simulink model "bicycle_drift_model"  (R2016a)
settings: Solver=VariableStepAuto  StartTime=0.0  StopTime=20  RelTol=1e-3
values from neighbouring files (symbols this model uses):
  a = 0.1    [setup.m]
  b = 0.155    [setup.m]
  C_alpha = 10    [setup.m]
  initial_states = [0 0 3]    [setup.m]
  Iz = 0.2    [setup.m]
  L = 0.255    [setup.m]    (also in veh_object2.m = obj_length)
  m = 5    [setup.m]
  mu = 0.2    [setup.m]
undefined symbols (not defined in the file): animation_update_interval, datetime, enable_CG_trace, enable_rearAxle_trace, plotAxisLimitMode, plotAxisLimits, save_anim_frames, vehicle_length, vehicle_width
settings Model: Creator=Cyrus  LastModifiedBy=Cyrus

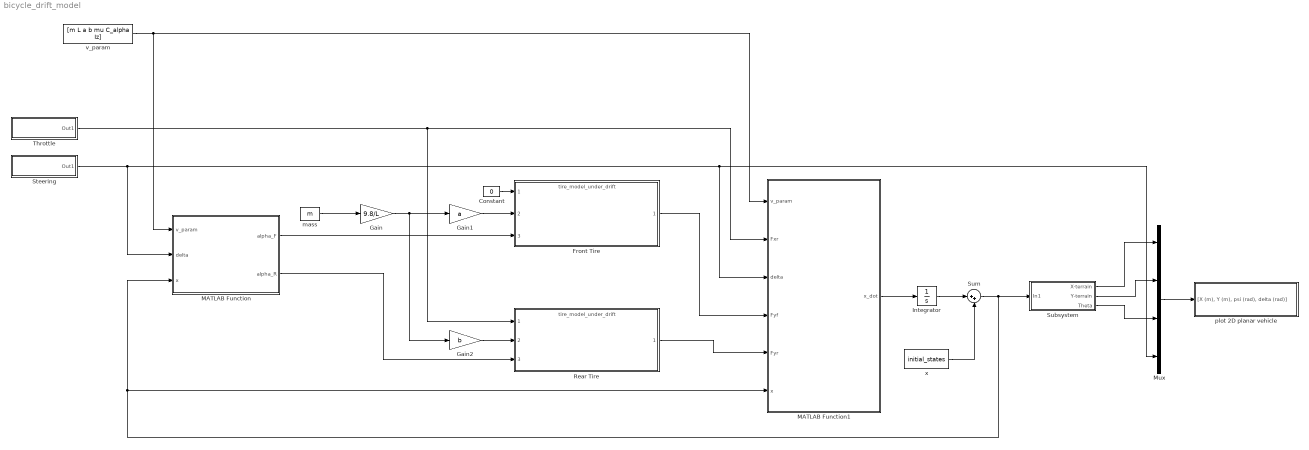
== system bicycle_drift_model ==
  Constant : Constant  Value=0
  Front Tire : ModelReference  ModelNameDialog=tire_model_under_drift.slx  SimulationMode=Normal  ModelReferenceVersion=1.21
  Gain : Gain  Gain=9.8/L
  Gain1 : Gain  Gain=a
  Gain2 : Gain  Gain=b
  Integrator : Integrator
  MATLAB Function : MATLAB Function  TreatAsAtomicUnit=on
  MATLAB Function1 : MATLAB Function  TreatAsAtomicUnit=on
  Mux : Mux
  Rear Tire : ModelReference  ModelNameDialog=tire_model_under_drift.slx  SimulationMode=Normal  ModelReferenceVersion=1.21
  Steering : Subsystem
  Subsystem : Subsystem
  Sum : Sum  Inputs=|++
  Throttle : Subsystem
  mass : Constant  Value=m
  plot 2D planar vehicle : Subsystem  mask(6DoF Animation){axisMode=plotAxisLimitMode, ax=plotAxisLimits, Ts=animation_update_interval, enable_CG_trace=enable_CG_trace, enable_rearAxle_trace=enable_rearAxle_trace, save_anim_frames=save_anim_frames, anim_frame_name_str=char(datetime('now','Format','yyyy-MM-dd_HH_mm_ss')), L=vehicle_length, W=vehicle_width}
      mask prompts: axisMode "Axis Mode (0->auto, 1->fixed, BOTH use Axes Limits below)"; ax "Axes limits [xmin xmax ymin ymax] (m):"; Ts "Time interval between updates (s):"; enable_CG_trace "Enable vehicle CG trace? (0/1)"; enable_rearAxle_trace "Enable rear axle trace? (0/1)"; save_anim_frames "Save animaton frames? (0/1)"; anim_frame_name_str "Animation sequence name (if save frames==1)"; L "Vehicle length (m)"; W "Vehicle width (m)"
      mask help:
      | Create a 2D animated view of a steering vehicle model with tires.
      |
      | Marc Compere
      | CompereM@saic.com
      | created : 22 August 2002
      | modified: 28 Dec 2015
      mask init:
      | Config.axisMode=axisMode;
      | Config.ax=ax;
      | Config.Ts=Ts;
      | Config.enable_CG_trace=enable_CG_trace;
      | Config.enable_rearAxle_trace=enable_rearAxle_trace;
      | Config.save_anim_frames=save_anim_frames;
      | Config.anim_frame_name_str=anim_frame_name_str;
      | Config.L=L;
      | Config.W=W;
      mask Help:
      | <p>This block generates a 3 dimensional display of a simulation trajectory, with the craft orientation displayed during flight</p>
      | 
      | <p>There are two inputs to this block, Position and Euler.  These inputs contain more than one signal as described below.</p>
      | 
      | <p><H4>Block Vector Input - Position</H4>
      | <ul>
      | <li>X Position</li>
      | <li>Y Position</li>
      | <li>Z Position</li>
      | </ul>
      | </p>
      | 
      | <p><H4>Block Vector Input - Euler</H4>
      |     <ul>
      |     <li>Roll Attitude</li>
      |     <li>Pitch Attitude</li>
      |     <li>Yaw Attitude</li>
      |    </ul>
      |    </p>
  v_param : Constant  Value=[m L a b mu C_alpha Iz]
  x : Constant  Value=initial_states
  wires:
  mass/1 -> Gain/1
  Gain1/1 -> Front Tire/2
  Gain2/1 -> Rear Tire/2
  MATLAB Function/1(alpha_F) -> Front Tire/3
  MATLAB Function/2(alpha_R) -> Rear Tire/3
  Gain/1 -> Gain2/1, Gain1/1
  Sum/1 -> MATLAB Function/3(x), MATLAB Function1/6(x), Subsystem/1(In1)
  MATLAB Function1/1(x_dot) -> Integrator/1
  Front Tire/1 -> MATLAB Function1/4(Fyf)
  Rear Tire/1 -> MATLAB Function1/5(Fyr)
  Throttle/1(Out1) -> Rear Tire/1, MATLAB Function1/2(Fxr)
  Constant/1 -> Front Tire/1
  Integrator/1 -> Sum/1
  x/1 -> Sum/2
  Steering/1(Out1) -> Mux/4, MATLAB Function1/3(delta), MATLAB Function/2(delta)
  Subsystem/1(X-terrain) -> Mux/1
  Subsystem/2(Y-terrain) -> Mux/2
  Subsystem/3("Theta ") -> Mux/3
  Mux/1 -> plot 2D planar vehicle/1("[X (m), Y (m), psi (rad), delta (rad)]")
  v_param/1 -> MATLAB Function1/1(v_param), MATLAB Function/1(v_param)

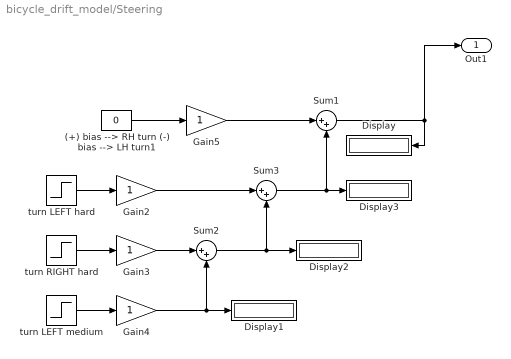
== system bicycle_drift_model/Steering ==
  (+) bias --> RH turn (-) bias --> LH turn1 : Constant  Value=0
  Display{,1..3} (4 alike) : Display
  Gain{2..5} (4 alike) : Gain
  Sum1 : Sum  Inputs=|++
  Sum2 : Sum  Inputs=|++
  Sum3 : Sum  Inputs=|++
  turn LEFT hard : Step  After=-0.5  SampleTime=0
  turn LEFT medium : Step  Time=11  After=-0.5  SampleTime=0
  turn RIGHT hard : Step  Time=6  After=+1  SampleTime=0
  Out1 : Outport
  wires:
  Sum1/1 -> Out1/1, Display/1
  (+) bias --> RH turn (-) bias --> LH turn1/1 -> Gain5/1
  turn RIGHT hard/1 -> Gain3/1
  turn LEFT medium/1 -> Gain4/1
  turn LEFT hard/1 -> Gain2/1
  Sum2/1 -> Display2/1, Sum3/2
  Sum3/1 -> Display3/1, Sum1/2
  Gain2/1 -> Sum3/1
  Gain3/1 -> Sum2/1
  Gain4/1 -> Display1/1, Sum2/2
  Gain5/1 -> Sum1/1

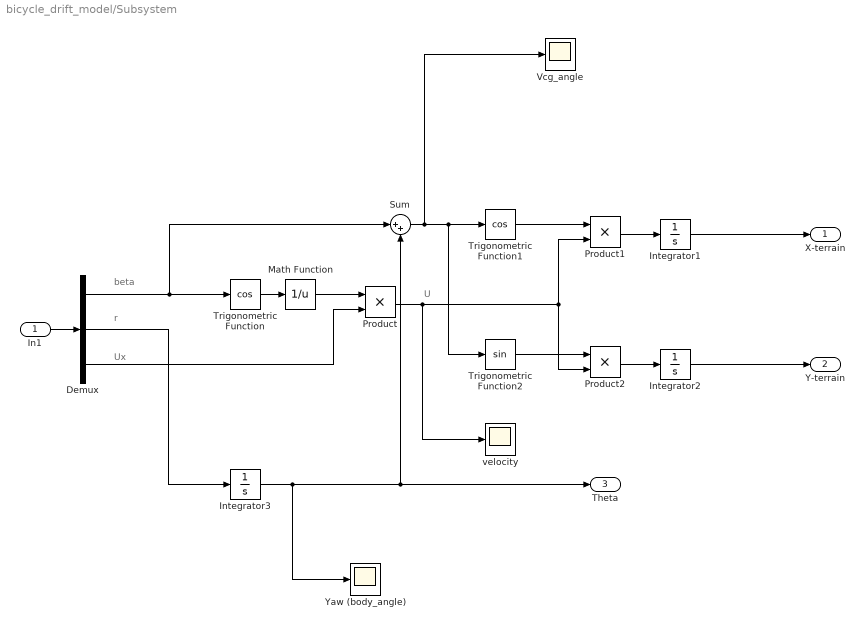
== system bicycle_drift_model/Subsystem ==
  note: U
  note: r
  note: Ux
  note: beta
  In1 : Inport
  Demux : Demux  Outputs=3
  Integrator1 : Integrator
  Integrator2 : Integrator
  Integrator3 : Integrator
  Math Function : Math  Operator=reciprocal  SaturateOnIntegerOverflow=on
  Product : Product
  Product1 : Product
  Product2 : Product
  Sum : Sum  Inputs=|++
  Trigonometric Function : Trigonometry  Operator=cos
  Trigonometric Function1 : Trigonometry  Operator=cos
  Trigonometric Function2 : Trigonometry
  Vcg_angle : Scope
  Yaw (body_angle) : Scope
  velocity : Scope
  X-terrain : Outport
  Y-terrain : Outport  Port=2
  "Theta " : Outport  Port=3
  wires:
  In1/1 -> Demux/1
  Demux/2 -> Integrator3/1
  Demux/3 -> Product/2
  Trigonometric Function/1 -> Math Function/1
  Math Function/1 -> Product/1
  Product/1 -> velocity/1, Product1/2, Product2/2
  Demux/1 -> Sum/1, Trigonometric Function/1
  Trigonometric Function1/1 -> Product1/1
  Trigonometric Function2/1 -> Product2/1
  Product1/1 -> Integrator1/1
  Product2/1 -> Integrator2/1
  Integrator1/1 -> X-terrain/1
  Integrator2/1 -> Y-terrain/1
  Integrator3/1 -> "Theta "/1, Sum/2, Yaw (body_angle)/1
  Sum/1 -> Vcg_angle/1, Trigonometric Function2/1, Trigonometric Function1/1

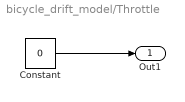
== system bicycle_drift_model/Throttle ==
  Constant : Constant  Value=0
  Out1 : Outport
  wires:
  Constant/1 -> Out1/1

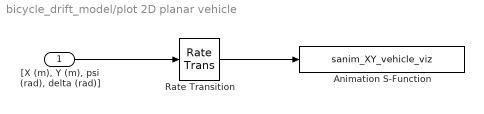
== system bicycle_drift_model/plot 2D planar vehicle ==
  "[X (m), Y (m), psi (rad), delta (rad)]" : Inport
  Animation S-Function : S-Function  FunctionName=sanim_XY_vehicle_viz  Parameters=Config  SFunctionDeploymentMode=off  EnableBusSupport=off
  Rate Transition : RateTransition  Integrity=off
  wires:
  "[X (m), Y (m), psi (rad), delta (rad)]"/1 -> Rate Transition/1
  Rate Transition/1 -> Animation S-Function/1

== matlab function bicycle_drift_model/MATLAB Function1 ==
  data: v_param input; Fxr input; delta input; Fyf input; Fyr input; x_dot output; x input
function x_dot = fcn(v_param,Fxr,delta,Fyf,Fyr,x)
%#codegen
m = v_param(1);
a = v_param(3);
b = v_param(4);
Iz = v_param(7);

beta = x(1);
r = x(2);
Ux = x(3);

beta_dot = (Fyf+Fyr)/(m*Ux)-r;
r_dot = (a*Fyf-b*Fyr)/Iz;
Ux_dot = (Fxr-Fyf*sin(delta))/m + r*Ux*beta;

x_dot = [beta_dot r_dot Ux_dot];

== matlab function bicycle_drift_model/MATLAB Function ==
  data: v_param input; delta input; x input; alpha_F output; alpha_R output
function [alpha_F, alpha_R] = fcn(v_param,delta,x)
%#codegen
a = v_param(3);
b = v_param(4);

beta = x(1);
r = x(2);
Ux = x(3);

alpha_F = atan(beta+(a/Ux)*r)-delta;
alpha_R = atan(beta-(b/Ux)*r);
